simulink model "Task_g"  (R2025b)
settings: Solver=VariableStepAuto  StartTime=0.0  StopTime=10000  RelTol=1e-3
model workspace (MAT data in the model file):
  F = [0.06  0  0; 0  0.06  0; 0  0  0]
values from neighbouring files (symbols this model uses):
  A = [ -(1/(R1*C1) + 1/(R2*C1)),   1/(R2*C1),                 0 ... (first row only)    [Lab_Prep.m]    (also in Lab_Session.m = [ -(k1 + k12),      k12,            0)
  B = [ kin1,   0 ... (first row only)    [Lab_Session.m]
  C = [0, 0, 1]    [Lab_Prep.m]    (also in Lab_Session.m = [0 0 1])
  D = [0 0]    [Lab_Session.m]
settings Model: Creator=DemoBox  LastModifiedBy=DemoBox

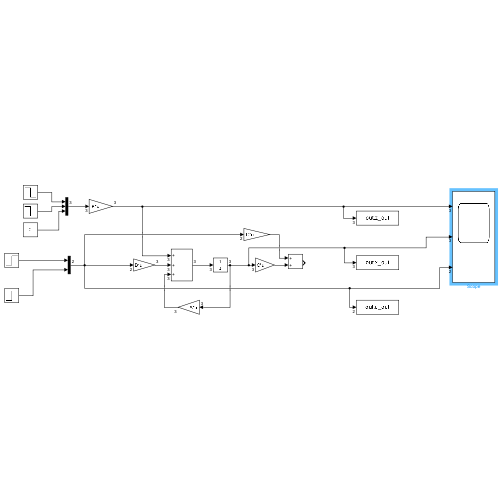
[thumbnail: Simulink's stored preview of the top-level diagram]
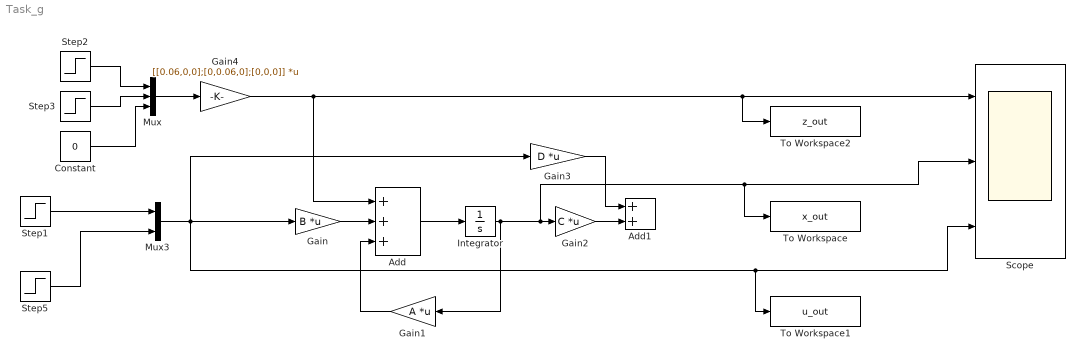
== system Task_g ==
  Add : Sum  Inputs=+++
  Add1 : Sum
  Constant : Constant  Value=0
  Gain : Gain  Gain=B  Multiplication=Matrix(K*u)
  Gain1 : Gain  Gain=A  Multiplication=Matrix(K*u)
  Gain2 : Gain  Gain=C  Multiplication=Matrix(K*u)
  Gain3 : Gain  Gain=D  Multiplication=Matrix(K*u)
  Gain4 : Gain  Gain=[[0.06,0,0];[0,0.06,0];[0,0,0]]  Multiplication=Matrix(K*u)
  Integrator : Integrator
  Mux : Mux  Inputs=3
  Mux3 : Mux  Inputs=2
  Scope : Scope  NumInputPorts=3
      settings: ActiveDisplayYMinimum=-0.077173880457346342  ActiveDisplayYMaximum=0.66456492411611723
  Step1 : Step  Time=0  After=0.1  SampleTime=0
  Step2 : Step  Time=4000  After=-0.02  SampleTime=0
  Step3 : Step  Time=6000  After=-0.05  SampleTime=0
  Step5 : Step  Time=0  After=0.1  SampleTime=0
  To Workspace : ToWorkspace  VariableName=x_out  SaveFormat=Timeseries  SampleTime=-1
  To Workspace1 : ToWorkspace  VariableName=u_out  SaveFormat=Timeseries  SampleTime=-1
  To Workspace2 : ToWorkspace  VariableName=z_out  SaveFormat=Timeseries  SampleTime=-1
  wires:
  Gain1/1 -> Add/3
  Gain/1 -> Add/2
  Add/1 -> Integrator/1
  Integrator/1 -> Gain1/1, Scope/2, To Workspace/1, Gain2/1
  Gain2/1 -> Add1/2
  Gain3/1 -> Add1/1
  Mux/1 -> Gain4/1
  Step2/1 -> Mux/1
  Step3/1 -> Mux/2
  Constant/1 -> Mux/3
  Gain4/1 -> Add/1, Scope/1, To Workspace2/1
  Mux3/1 -> Gain3/1, To Workspace1/1, Scope/3, Gain/1
  Step1/1 -> Mux3/1
  Step5/1 -> Mux3/2
